simulink model "MGietka_2cd"  (R2020b)
settings: Solver=VariableStepAuto  StartTime=0.0  StopTime=10.0  RelTol=1e-3
undefined symbols (not defined in the file): A, B, C, N
settings Model: Creator=Mati  LastModifiedBy=Mati

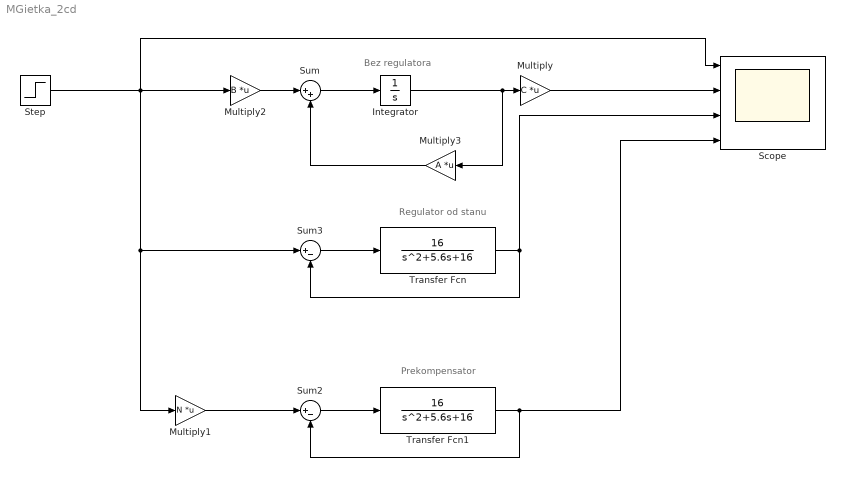
== system MGietka_2cd ==
  note: Prekompensator
  note: Regulator od stanu
  note: Bez regulatora
  Integrator : Integrator
  Multiply : Gain  Gain=C  Multiplication=Matrix(K*u)
  Multiply1 : Gain  Gain=N  Multiplication=Matrix(K*u)
  Multiply2 : Gain  Gain=B  Multiplication=Matrix(K*u)
  Multiply3 : Gain  Gain=A  Multiplication=Matrix(K*u)
  Scope : Scope  NumInputPorts=4
  Step : Step  SampleTime=0
  Sum : Sum  Inputs=|++
  Sum2 : Sum  Inputs=|+-
  Sum3 : Sum  Inputs=|+-
  Transfer Fcn : TransferFcn  Numerator=16  Denominator=[1 5.6 16]
  Transfer Fcn1 : TransferFcn  Numerator=16  Denominator=[1 5.6 16]
  wires:
  Sum/1 -> Integrator/1
  Integrator/1 -> Multiply3/1, Multiply/1
  Multiply2/1 -> Sum/1
  Multiply3/1 -> Sum/2
  Step/1 -> Multiply1/1, Sum3/1, Scope/1, Multiply2/1
  Sum3/1 -> Transfer Fcn/1
  Multiply1/1 -> Sum2/1
  Sum2/1 -> Transfer Fcn1/1
  Multiply/1 -> Scope/2
  Transfer Fcn1/1 -> Scope/4, Sum2/2
  Transfer Fcn/1 -> Sum3/2, Scope/3
